simulink model "HDL_source"  (R2019a)
settings: Solver=FixedStepDiscrete  StartTime=0.0  StopTime=0.1  RelTol=1e-3
PreLoadFcn:
  | load('visionhdlLaneDetectionInit.mat');
  | 
  | %Birds-Eye View Parameters:
  | T_unreal = [-0.346719845290643,-3.45626583672944e-16,-2.42608110520569e-19;-1.76272742794994,-2.62399506819665,-0.00185184300876343;1283.14845282490,1569.57420684550,1];
  | shiftleft = single([-5,-5,-5,-5,-5,-5,-5,-5,-5,-5,   -5,-4,-2,-2,-2,-2,0,0,0,1,    1,2,3,4,5,6,7,10,11,13,     15,17,20,22,26,30,33,38,42,46]);
  | shiftright = single([-20,-20,-20,-20,-20,-20,-20,-20,-20,-20,    -20,-20,-20,-21,-22,-23,-24,-24,-24,-25,    -26,-27,-28,-29,-30,-32,-33,-35,-37,-39,    -41,-45,-46,-50,-53,-57,-61,-67,-72,-78]);
StartFcn:
  | warning('off','Coder:MATLAB:polyfit_RepeatedPointsOrRescale');
  | warning('off','Coder:MATLAB:rankDeficientMatrix');
StopFcn:
  | warning('on','Coder:MATLAB:polyfit_RepeatedPointsOrRescale');
  | warning('on','Coder:MATLAB:rankDeficientMatrix');
undefined symbols (not defined in the file): gray, h1, imresize, Rec, SDTV
libraries: simulink x31, hdlsllib x19, visionhdlutilities x6, visionhdlstatistics x4, visiongeotforms x3, visionhdlio x2, visiontextngfix x2, visionhdlconversions x1, visionhdlgeotforms x1, visionhdlfilter x1, dspvision x1, visionsinks x1
(part 3 of 3)

== matlab function HDL_source/SWLaneFitandOverlay/FitLanesAndOverlay/FitLanes/FitLeftPolyLane ==
  data: laneCIn input; P output
function P  = fitLane(laneCIn)

%#codegen

persistent P1;
if isempty(P1)
    P1 = [0 0 0];
end

% laneC = zeros(40,2);
inliersMask = zeros(1,100);
inlierTable1 = zeros(2,100);
P1T= single([0 0 0]);
% % aviod using sortrows (time complexity O(nlogn))
% % now O(n) oeprations
laneC = single(zeros(40,2));
 numG = 0;
 for jj = 1:1:40
     if(laneCIn(jj,1)>1)
         numG = numG+1;
         laneC(numG,1:2) = single(laneCIn(jj,1:2));
     end
 end


% ignore when inliers/total < curInliersRatio
curInliersRatio = 0.4;

% inlierIndex1-1 = num of inliers in best model
% is also used to determine whether a best model is found
inlierIndex1 = 0;

% K = log(1-P)/log(1-w^s)
K = 70; % max iteration

distanceMax = 67; % distance Threshold

curvatureMax = 0.003; % curvature Threshold for P(1); maybe removed for curved lanes


if numG>3
    
    %%% Use RANSAC for robust fit of 2nd order polynomial
    
    for ii = 1:1:K

        a = randperm(numG,3);
        
        P1T = polyfit(laneC(a,2), laneC(a,1),2);
        
        % O(n) operations
        numInliers = 0;
        for jj = 1:1:numG
            x1 = floor(polyval(P1T,laneC(jj,1)));
            inliersMask(jj) = abs(x1-laneC(jj,1))<distanceMax;
            if(inliersMask(jj))
                numInliers = numInliers + 1;
            end
        end

        if ((numInliers/numG)>curInliersRatio && abs(P1T(1))<curvatureMax && numInliers>2)
            % record the inliers for current best model  
            curInliersRatio = numInliers/numG;
            inlierIndex1 = 1;
            for jj = 1:1:numG
                if(inliersMask(jj))
                    inlierTable1(1,inlierIndex1) = laneC(jj,2);
                    inlierTable1(2,inlierIndex1) = laneC(jj,1);
                    inlierIndex1 = inlierIndex1 + 1;
                end
            end
        end
        
    end
  
end

    P1T = polyfit(inlierTable1(1,1:inlierIndex1-1), inlierTable1(2,1:inlierIndex1-1),2);


if abs(P1T(1))<curvatureMax % if found a best model; initial inlierIndex1 = 0;
    % refine the fitted line using all inliers
    P1 = P1T;
end

P = P1;

== matlab function HDL_source/SWLaneFitandOverlay/FitLanesAndOverlay/FitLanes/FitRightPolyLane ==
  data: laneCIn input; P output
function P  = fitLane(laneCIn)

%#codegen

persistent P1;
if isempty(P1)
    P1 = [0 0 0];
end

% laneC = zeros(40,2);
inliersMask = zeros(1,100);
inlierTable1 = zeros(2,100);
P1T= single([0 0 0]);
% % aviod using sortrows (time complexity O(nlogn))
% % now O(n) oeprations
laneC = single(zeros(40,2));
 numG = 0;
 for jj = 1:1:40
     if(laneCIn(jj,1)>1)
         numG = numG+1;
         laneC(numG,1:2) = single(laneCIn(jj,1:2));
     end
 end


% ignore when inliers/total < curInliersRatio
curInliersRatio = 0.4;

% inlierIndex1-1 = num of inliers in best model
% is also used to determine whether a best model is found
inlierIndex1 = 0;

% K = log(1-P)/log(1-w^s)
K = 70; % max iteration

distanceMax = 67; % distance Threshold

curvatureMax = 0.003; % curvature Threshold for P(1); maybe removed for curved lanes


if numG>3
    
    %%% Use RANSAC for robust fit of 2nd order polynomial
    
    for ii = 1:1:K

        a = randperm(numG,3);
        
        P1T = polyfit(laneC(a,2), laneC(a,1),2);
        
        % O(n) operations
        numInliers = 0;
        for jj = 1:1:numG
            x1 = floor(polyval(P1T,laneC(jj,1)));
            inliersMask(jj) = abs(x1-laneC(jj,1))<distanceMax;
            if(inliersMask(jj))
                numInliers = numInliers + 1;
            end
        end

        if ((numInliers/numG)>curInliersRatio && abs(P1T(1))<curvatureMax && numInliers>2)
            % record the inliers for current best model  
            curInliersRatio = numInliers/numG;
            inlierIndex1 = 1;
            for jj = 1:1:numG
                if(inliersMask(jj))
                    inlierTable1(1,inlierIndex1) = laneC(jj,2);
                    inlierTable1(2,inlierIndex1) = laneC(jj,1);
                    inlierIndex1 = inlierIndex1 + 1;
                end
            end
        end
        
    end
  
end

    P1T = polyfit(inlierTable1(1,1:inlierIndex1-1), inlierTable1(2,1:inlierIndex1-1),2);


if abs(P1T(1))<curvatureMax % if found a best model; initial inlierIndex1 = 0;
    % refine the fitted line using all inliers
    P1 = P1T;
end

P = P1;

== matlab function HDL_source/SWLaneFitandOverlay/FitLanesAndOverlay/OverlayLaneMarkings/DrawPolynomial ==
  data: P1 input; Im output; Im input
function Im  = DrawLane(P1,Im)
%#codegen

% ipmImage = uint8(zeros(900,640,3));
% HD: uint8(zeros(1575,1440,3));
RGBVal = [0,255,9];



  for ii = 1:1:1080
      x1E = floor(polyval(P1,ii));
      
      if x1E <=5 || isnan(x1E)
          x1E = 6;
      elseif x1E>=1919
          x1E=1919;
      end
      
 
      Im(ii,x1E+0,:) = RGBVal;
      Im(ii,x1E-1,:) = RGBVal;
      Im(ii,x1E-2,:) = RGBVal;
      Im(ii,x1E-3,:) = RGBVal;
      Im(ii,x1E-4,:) = RGBVal;
      Im(ii,x1E-5,:) = RGBVal;

      
      
  end


% Im = ipmImage;

== matlab function HDL_source/SWLaneFitandOverlay/FitLanesAndOverlay/OverlayLaneMarkings/OverlayPolynomialLane1 ==
  data: P1 input; Im output; Im input
function Im  = fcn(P1,Im)
%#codegen

% ipmImage = uint8(zeros(900,640,3));
% HD: uint8(zeros(1575,1440,3));
RGBVal = [0,255,9];



  for ii = 1:1:1080
      x1E = floor(polyval(P1,ii));
      
      if x1E <=50 || isnan(x1E)
          x1E = 6;
      elseif x1E>=1919
          x1E=1919;
      end
      
 
      Im(ii,x1E+0,:) = RGBVal;
      Im(ii,x1E-1,:) = RGBVal;
      Im(ii,x1E-2,:) = RGBVal;
      Im(ii,x1E-3,:) = RGBVal;
      Im(ii,x1E-4,:) = RGBVal;
      Im(ii,x1E-5,:) = RGBVal;

      
      
  end


% Im = ipmImage;

== matlab function HDL_source/FPGALaneDetection/Lane Detection Algorithm/CtrlInterface1 ==
  data: LaneLeftin input; LaneRightin input; enable input; hwStart input; LaneLeftout output; LaneRightout output; hwDone input; dataReady output; swStart input
function [LaneLeftout, LaneRightout, dataReady] = fcn(LaneLeftin, LaneRightin, enable, hwStart, hwDone, swStart)

persistent regLaneLeft;
persistent regLaneRight;
persistent FSMState;

% define states
S0 = uint8(0);
S1 = uint8(1);
S2 = uint8(2);

if isempty(regLaneLeft)
   regLaneLeft = zeros(1,40,'uint16');
end

if isempty(regLaneRight)
   regLaneRight = zeros(1,40,'uint16');
end

if isempty(FSMState)
   FSMState = S0; 
end

switch FSMState
    case S0 %Wait for SW and HW to be ready
        dataReady =  false;
        
        if swStart && hwStart
            FSMState = S1;
        else
            FSMState = S0;
        end
        
    case S1 %buffer vectors
        dataReady =  false;
        
        if(enable)
        regLaneLeft(1:40) = [regLaneLeft(2:40),LaneLeftin];
        regLaneRight(1:40) = [regLaneRight(2:40),LaneRightin];
        end

        if hwDone
            FSMState = S2;
        else
            FSMState = S1;
        end
          
    case S2 % wait for sw ack (sw ready low)
        dataReady =  true;
        
        if ~swStart
            FSMState = S0;
        else
            FSMState = S2;
        end
        
    otherwise
        dataReady =  false;
        FSMState = S0;
end

LaneLeftout = regLaneLeft';
LaneRightout = regLaneRight';

end
